simulink model "stewartpid_simulink"  (R2021b)
settings: Solver=FixedStepAuto  StartTime=0.0  StopTime=10.0  FixedStep=0.001  RelTol=1e-3
values from neighbouring files (symbols this model uses):
  contact = 0.05    [runthis.m]
  downMass = 0.1    [runthis.m]
  Kd = 0    [runthis.m]
  Ki = 0    [runthis.m]
  Kp = 0    [runthis.m]
  l1 = 0.35    [runthis.m]
  upMass = 0.1    [runthis.m]
undefined symbols (not defined in the file or in its folder): X, Y, Z
libraries: sm_lib x96, nesl_utility x30, slpidlib x1, sharedtransform x1
(part 1 of 3)
settings Model: Creator=Hitsz  LastModifiedBy=Hitsz

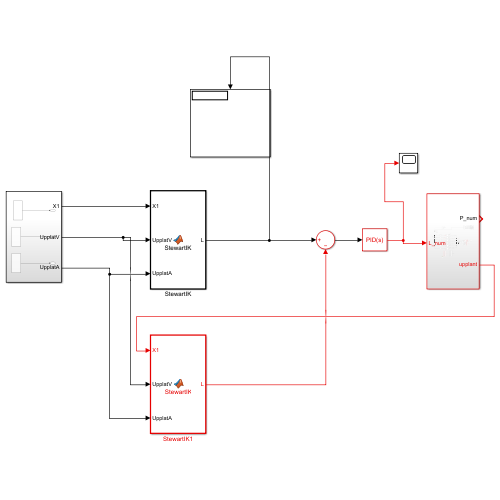
[thumbnail: Simulink's stored preview of the top-level diagram]
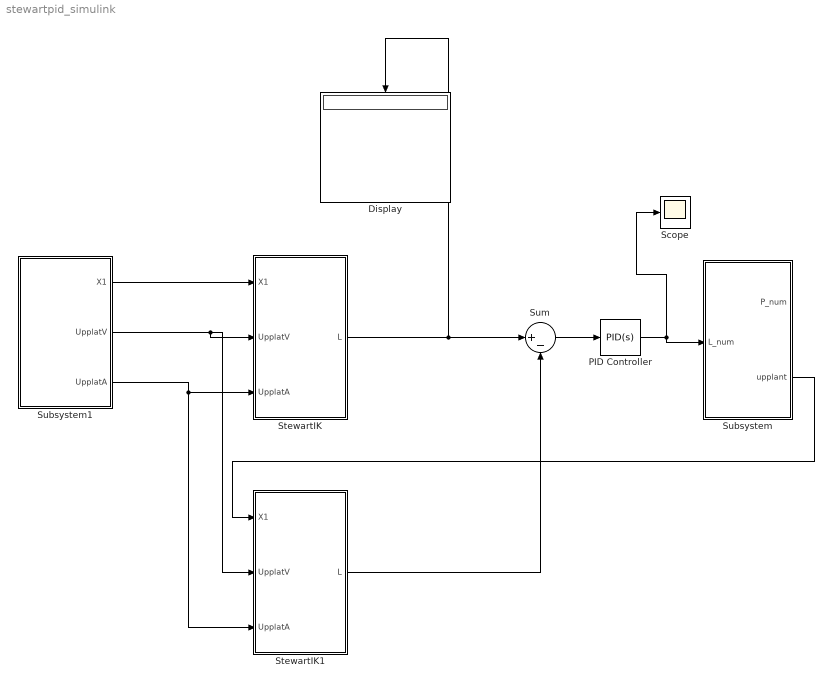
== system stewartpid_simulink ==
  Display : Display
  PID Controller : slpidlib/PID Controller  Controller=PID  Form=Parallel  TimeDomain=Continuous-time  UseExternalTs=off  SampleTime=-1  IntegratorMethod=Forward Euler  FilterMethod=Forward Euler  ControllerParametersSource=internal  P=Kp  I=Ki  D=Kd  UseFilter=on  N=100  TunerSelectOption=Transfer Function Based (PID Tuner App)  InitialConditionSource=internal  InitialConditionForIntegrator=0  InitialConditionForFilter=0  DifferentiatorICPrevScaledInput=0  ExternalReset=none  TrackingMode=off  Kt=1  LimitOutput=off  SatLimitsSource=internal  UpperSaturationLimit=inf  LowerSaturationLimit=-inf  LinearizeAsGain=on  AntiWindupMode=none  Kb=1  POutMin=[]  POutMax=[]  IOutMin=[]  IOutMax=[]  DOutMin=[]  DOutMax=[]  NOutMin=[]  NOutMax=[]  SumOutMin=[]  SumOutMax=[]  SaturationOutMin=[]  SaturationOutMax=[]  PParamMin=[]  PParamMax=[]  IParamMin=[]  IParamMax=[]  DParamMin=[]  DParamMax=[]  NParamMin=[]  NParamMax=[]  KbParamMin=[]  KbParamMax=[]  KtParamMin=[]  KtParamMax=[]  KbOutMin=[]  KbOutMax=[]  KtOutMin=[]  KtOutMax=[]  IntegratorOutMin=[]  IntegratorOutMax=[]  FilterOutMin=[]  FilterOutMax=[]  SumI1OutMin=[]  SumI1OutMax=[]  SumI2OutMin=[]  SumI2OutMax=[]  SumI3OutMin=[]  SumI3OutMax=[]  SumI4OutMin=[]  SumI4OutMax=[]  SumDOutMin=[]  SumDOutMax=[]  DifferentiatorOutMin=[]  DifferentiatorOutMax=[]  FilterDiffOutCoefMin=[]  FilterDiffOutCoefMax=[]  ReciprocalOutMin=[]  ReciprocalOutMax=[]  SumDenOutMin=[]  SumDenOutMax=[]  SumNumOutMin=[]  SumNumOutMax=[]  DivideOutMin=[]  DivideOutMax=[]  UdiffTsProdOutMin=[]  UdiffTsProdOutMax=[]  NTsProdOutMin=[]  NTsProdOutMax=[]  UintegralTsProdOutMin=[]  UintegralTsProdOutMax=[]  UngainTsProdOutMin=[]  UngainTsProdOutMax=[]  IntegratorContinuousStateAttributes=''  IntegratorStateMustResolveToSignalObject=off  IntegratorRTWStateStorageClass=Auto  FilterContinuousStateAttributes=''  FilterStateMustResolveToSignalObject=off  FilterRTWStateStorageClass=Auto  ParallelPVariant=InternalParameters  IdealPVariant=Disabled  IVariant=InternalParameters  DVariant=InternalParameters  IntegratorVariant=Continuous  SatVariant=Disabled  AWVariant=Passthrough  PCopyVariant=Disabled  TRVariant=Disabled  FdbkBlocksVariant=Forward  IdealPFdbkVariant=Disabled  SatFdbkVariant=Disabled  DerivativeFilterVariant=ContFilter  NVariant=InternalParameters  NCopyVariant=Disabled  FilterICVariant=InternalICsFilter  IntegratorICVariant=InternalICs  ExternalResetVariant=Disabled  TRSumVariant=Passthrough  SumFdbkVariant=Disabled  SumVariant=Sum_PID  TsampFilterVariant=InternalTs  TsampNgainVariant=Passthrough  TsampIntegralVariant=Passthrough  ExternalSaturationOutDataTypeStr=Inherit: Same as second input
  Scope : Scope
  StewartIK : MATLAB Function  TreatAsAtomicUnit=on
  StewartIK1 : MATLAB Function  TreatAsAtomicUnit=on
  Subsystem : Subsystem
  Subsystem1 : Subsystem
  Sum : Sum  Inputs=|+-
  wires:
  Subsystem1/1(X1) -> StewartIK/1(X1)
  Subsystem1/2(UpplatV) -> StewartIK1/2(UpplatV), StewartIK/2(UpplatV)
  Subsystem1/3(UpplatA) -> StewartIK1/3(UpplatA), StewartIK/3(UpplatA)
  StewartIK/1(L) -> Sum/1, Display/1
  Sum/1 -> PID Controller/1
  PID Controller/1 -> Scope/1, Subsystem/1(L_num)
  Subsystem/2(upplant) -> StewartIK1/1(X1)
  StewartIK1/1(L) -> Sum/2

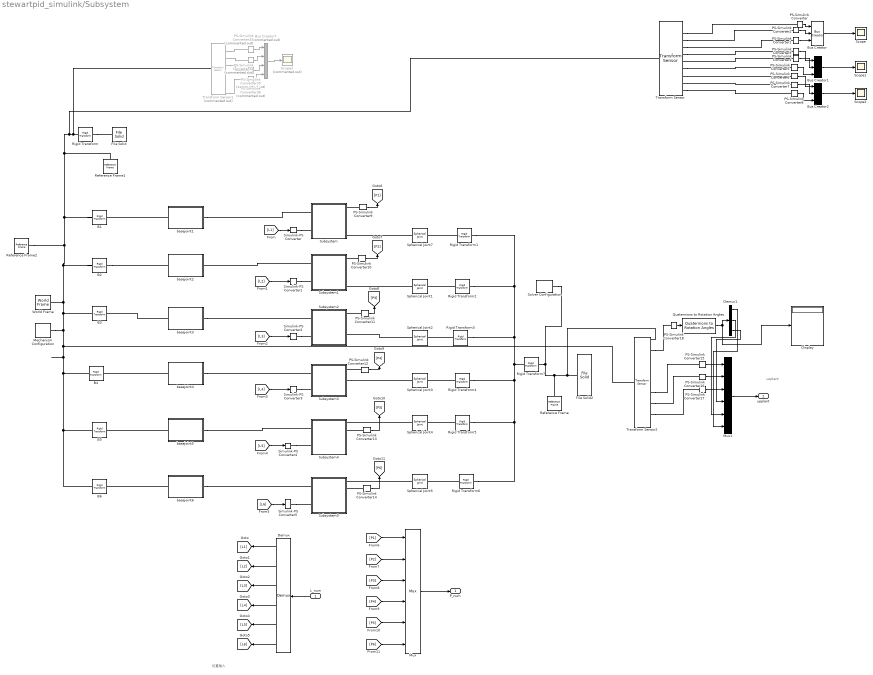
== system stewartpid_simulink/Subsystem ==
  note: uoplant
  note: 位置输入
  L_num : Inport
  "B1 " : sm_lib/Frames and Transforms/Rigid Transform  TranslationMethod=Cartesian  TranslationStandardOffset=0  TranslationLengthUnit=m  TranslationStandardAxis=+Z  TranslationCartesianOffset=B1  TranslationROffset=0  TranslationROffsetUnits=m  TranslationZOffset=0  TranslationZOffsetUnits=m  TranslationThetaOffset=0  TranslationThetaOffsetUnits=deg  RotationMethod=None  RotationAngleUnits=deg  RotationStandardAxis=+Z  RotationAngle=0.0  RotationArbitraryAxis=[0 0 1]  FollAlignAxisA=+X  BaseAlignAxisA=+Y  FollAlignAxisB=+Y  BaseAlignAxisB=+Z  RotationSequenceAxes=FollowerAxes  RotationSequence=XYX  RotationSequenceAngles=[0 0 0]  RotationSequenceAnglesUnits=deg  RotationMatrix=[1 0 0; 0 1 0; 0 0 1]
  "B2 " : sm_lib/Frames and Transforms/Rigid Transform  TranslationMethod=Cartesian  TranslationStandardOffset=0  TranslationLengthUnit=m  TranslationStandardAxis=+Z  TranslationCartesianOffset=B2  TranslationROffset=0  TranslationROffsetUnits=m  TranslationZOffset=0  TranslationZOffsetUnits=m  TranslationThetaOffset=0  TranslationThetaOffsetUnits=deg  RotationMethod=None  RotationAngleUnits=deg  RotationStandardAxis=+Z  RotationAngle=0.0  RotationArbitraryAxis=[0 0 1]  FollAlignAxisA=+X  BaseAlignAxisA=+Y  FollAlignAxisB=+Y  BaseAlignAxisB=+Z  RotationSequenceAxes=FollowerAxes  RotationSequence=XYX  RotationSequenceAngles=[0 0 0]  RotationSequenceAnglesUnits=deg  RotationMatrix=[1 0 0; 0 1 0; 0 0 1]
  "B3 " : sm_lib/Frames and Transforms/Rigid Transform  TranslationMethod=Cartesian  TranslationStandardOffset=0  TranslationLengthUnit=m  TranslationStandardAxis=+Z  TranslationCartesianOffset=B3  TranslationROffset=0  TranslationROffsetUnits=m  TranslationZOffset=0  TranslationZOffsetUnits=m  TranslationThetaOffset=0  TranslationThetaOffsetUnits=deg  RotationMethod=None  RotationAngleUnits=deg  RotationStandardAxis=+Z  RotationAngle=0.0  RotationArbitraryAxis=[0 0 1]  FollAlignAxisA=+X  BaseAlignAxisA=+Y  FollAlignAxisB=+Y  BaseAlignAxisB=+Z  RotationSequenceAxes=FollowerAxes  RotationSequence=XYX  RotationSequenceAngles=[0 0 0]  RotationSequenceAnglesUnits=deg  RotationMatrix=[1 0 0; 0 1 0; 0 0 1]
  "B4 " : sm_lib/Frames and Transforms/Rigid Transform  TranslationMethod=Cartesian  TranslationStandardOffset=0  TranslationLengthUnit=m  TranslationStandardAxis=+Z  TranslationCartesianOffset=B4  TranslationROffset=0  TranslationROffsetUnits=m  TranslationZOffset=0  TranslationZOffsetUnits=m  TranslationThetaOffset=0  TranslationThetaOffsetUnits=deg  RotationMethod=None  RotationAngleUnits=deg  RotationStandardAxis=+Z  RotationAngle=0.0  RotationArbitraryAxis=[0 0 1]  FollAlignAxisA=+X  BaseAlignAxisA=+Y  FollAlignAxisB=+Y  BaseAlignAxisB=+Z  RotationSequenceAxes=FollowerAxes  RotationSequence=XYX  RotationSequenceAngles=[0 0 0]  RotationSequenceAnglesUnits=deg  RotationMatrix=[1 0 0; 0 1 0; 0 0 1]
  "B5 " : sm_lib/Frames and Transforms/Rigid Transform  TranslationMethod=Cartesian  TranslationStandardOffset=0  TranslationLengthUnit=m  TranslationStandardAxis=+Z  TranslationCartesianOffset=B5  TranslationROffset=0  TranslationROffsetUnits=m  TranslationZOffset=0  TranslationZOffsetUnits=m  TranslationThetaOffset=0  TranslationThetaOffsetUnits=deg  RotationMethod=None  RotationAngleUnits=deg  RotationStandardAxis=+Z  RotationAngle=0.0  RotationArbitraryAxis=[0 0 1]  FollAlignAxisA=+X  BaseAlignAxisA=+Y  FollAlignAxisB=+Y  BaseAlignAxisB=+Z  RotationSequenceAxes=FollowerAxes  RotationSequence=XYX  RotationSequenceAngles=[0 0 0]  RotationSequenceAnglesUnits=deg  RotationMatrix=[1 0 0; 0 1 0; 0 0 1]
  "B6 " : sm_lib/Frames and Transforms/Rigid Transform  TranslationMethod=Cartesian  TranslationStandardOffset=0  TranslationLengthUnit=m  TranslationStandardAxis=+Z  TranslationCartesianOffset=B6  TranslationROffset=0  TranslationROffsetUnits=m  TranslationZOffset=0  TranslationZOffsetUnits=m  TranslationThetaOffset=0  TranslationThetaOffsetUnits=deg  RotationMethod=None  RotationAngleUnits=deg  RotationStandardAxis=+Z  RotationAngle=0.0  RotationArbitraryAxis=[0 0 1]  FollAlignAxisA=+X  BaseAlignAxisA=+Y  FollAlignAxisB=+Y  BaseAlignAxisB=+Z  RotationSequenceAxes=FollowerAxes  RotationSequence=XYX  RotationSequenceAngles=[0 0 0]  RotationSequenceAnglesUnits=deg  RotationMatrix=[1 0 0; 0 1 0; 0 0 1]
  Bus Creator : BusCreator  Inputs=3
  Bus Creator1 : BusCreator  Inputs=3
  Bus Creator2 : BusCreator  Inputs=3
  Bus Creator7 : BusCreator  Commented=on  Inputs=4
  Demux : Demux  Outputs=6
  Demux1 : Demux  Outputs=3
  Display : Display
  File Solid : sm_lib/Body Elements/File Solid  ExtGeomFileName=E:\onedrive\stewart_system\3_6_redundant\matlab_code\verification\verificationWithTraditionalControl\DOWN.STEP  UnitType=FromFile  ExtGeomFileUnits=m  StepReaderType=HEX  ExportConvexHullGeometry=off  InertiaType=Custom  Mass=1  MassUnits=kg  CenterOfMass=[0 0 0]  CenterOfMassUnits=m  MomentsOfInertia=[1 1 1]  MomentsOfInertiaUnits=kg*m^2  ProductsOfInertia=[0 0 0]  ProductsOfInertiaUnits=kg*m^2  BasedOnType=DensityFromFile  Density=1000  DensityUnits=kg/m^3  DoExposeReferenceFrame=off  SerializedFrames=<Frames><Frame><Id>Frame1</Id><Value><Name>F1</Name><Origin><Source>ReferenceFrame</Source><FeatureName></FeatureName></Origin><PrimaryAxis><DefinedDirection>+Z</DefinedDirection><Source>ReferenceFrame</Source><SourceDirection>+Z</SourceDirection><FeatureName></FeatureName></PrimaryAxis><SecondaryAxis><DefinedDirection>+X</DefinedDirection><Source>ReferenceFrame</Source><SourceDirection>+X</SourceDirection><FeatureName></FeatureName></SecondaryAxis></Value></Frame></Frames>  GraphicType=FromGeometry  MarkerShape=Sphere  MarkerSize=10  GraphicVisPropType=SimpleVisualProperties  GraphicDiffuseColor=[0.8 0.8 0.0]  GraphicSpecularColor=[0.5 0.5 0.5 1.0]  GraphicAmbientColor=[0.15 0.15 0.15 1.0]  GraphicEmissiveColor=[0.0 0.0 0.0 1.0]  GraphicShininess=75  GraphicOpacity=1.0
  File Solid2 : sm_lib/Body Elements/File Solid  ExtGeomFileName=E:\onedrive\stewart_system\3_6_redundant\matlab_code\verification\verificationWithTraditionalControl\UP.STEP  UnitType=FromFile  ExtGeomFileUnits=m  StepReaderType=HEX  ExportConvexHullGeometry=off  InertiaType=Custom  Mass=1.5  MassUnits=kg  CenterOfMass=[0 0 0]  CenterOfMassUnits=m  MomentsOfInertia=[0.08 0.08 .08]  MomentsOfInertiaUnits=kg*m^2  ProductsOfInertia=[0 0 0]  ProductsOfInertiaUnits=kg*m^2  BasedOnType=DensityFromFile  Density=1000  DensityUnits=kg/m^3  DoExposeReferenceFrame=off  SerializedFrames=<Frames><Frame><Id>Frame1</Id><Value><Name>M0</Name><Origin><Source>ReferenceFrame</Source><FeatureName></FeatureName></Origin><PrimaryAxis><DefinedDirection>+Z</DefinedDirection><Source>ReferenceFrame</Source><SourceDirection>+Z</SourceDirection><FeatureName></FeatureName></PrimaryAxis><SecondaryAxis><DefinedDirection>+X</DefinedDirection><Source>ReferenceFrame</Source><SourceDirection>+X</SourceDirection><FeatureName></FeatureName></SecondaryAxis></Value></Frame></Frames>  GraphicType=FromGeometry  MarkerShape=Sphere  MarkerSize=10  GraphicVisPropType=SimpleVisualProperties  GraphicDiffuseColor=[1.0 0.0 0.8]  GraphicSpecularColor=[0.5 0.5 0.5 1.0]  GraphicAmbientColor=[0.15 0.15 0.15 1.0]  GraphicEmissiveColor=[0.0 0.0 0.0 1.0]  GraphicShininess=75  GraphicOpacity=1.0
  Mechanism Configuration : sm_lib/Utilities/Mechanism Configuration  UniformGravity=Constant  GravityVector=[0 0 -9.807]  GravityUnits=m/s^2  LinearizationDelta=0.001  JointModeTransitionNonlinearIterations=2
  Mux : Mux  Inputs=6
  Mux1 : Mux  Inputs=6
  PS-Simulink Converter{,1..18} (19 alike) : nesl_utility/PS-Simulink Converter  PhysicalDomain=network_engine_domain  SubClassName=ps_output  LeftPortType=input  RightPortType=output  PseudoPeriodic=off  Frequencies=[]  Unit=inherit  AffineConversion=off
      settings: SourceProductBaseCode=PW,SS
  PS-Simulink Converter{33..36} (4 alike) : nesl_utility/PS-Simulink Converter  Commented=on  PhysicalDomain=network_engine_domain  SubClassName=ps_output  LeftPortType=input  RightPortType=output  PseudoPeriodic=off  Frequencies=[]  Unit=inherit  AffineConversion=off
      settings: SourceProductBaseCode=PW,SS
  Quaternions to Rotation Angles : sharedtransform/Quaternions to Rotation Angles  rotationOrder=ZYX  aMode=aMode
      settings: SourceProductBaseCode=AE,PW,DR,MT,UV,VE
  Reference Frame : sm_lib/Frames and Transforms/Reference Frame
  Reference Frame1 : sm_lib/Frames and Transforms/Reference Frame
  Reference Frame2 : sm_lib/Frames and Transforms/Reference Frame
  Rigid Transform : sm_lib/Frames and Transforms/Rigid Transform  TranslationMethod=None  TranslationStandardOffset=0  TranslationLengthUnit=m  TranslationStandardAxis=+Z  TranslationCartesianOffset=[0 0 0]  TranslationROffset=0  TranslationROffsetUnits=m  TranslationZOffset=0  TranslationZOffsetUnits=m  TranslationThetaOffset=0  TranslationThetaOffsetUnits=deg  RotationMethod=None  RotationAngleUnits=deg  RotationStandardAxis=+X  RotationAngle=90  RotationArbitraryAxis=[0 0 1]  FollAlignAxisA=+X  BaseAlignAxisA=+Y  FollAlignAxisB=+Y  BaseAlignAxisB=+Z  RotationSequenceAxes=FollowerAxes  RotationSequence=XYX  RotationSequenceAngles=[0 0 0]  RotationSequenceAnglesUnits=deg  RotationMatrix=[1 0 0; 0 1 0; 0 0 1]
  Rigid Transform1 : sm_lib/Frames and Transforms/Rigid Transform  TranslationMethod=Cartesian  TranslationStandardOffset=0  TranslationLengthUnit=m  TranslationStandardAxis=+Z  TranslationCartesianOffset=T1_Ti  TranslationROffset=0  TranslationROffsetUnits=m  TranslationZOffset=0  TranslationZOffsetUnits=m  TranslationThetaOffset=0  TranslationThetaOffsetUnits=deg  RotationMethod=None  RotationAngleUnits=deg  RotationStandardAxis=+Z  RotationAngle=0.0  RotationArbitraryAxis=[0 0 1]  FollAlignAxisA=+X  BaseAlignAxisA=+Y  FollAlignAxisB=+Y  BaseAlignAxisB=+Z  RotationSequenceAxes=FollowerAxes  RotationSequence=XYX  RotationSequenceAngles=[0 0 0]  RotationSequenceAnglesUnits=deg  RotationMatrix=[1 0 0; 0 1 0; 0 0 1]
  Rigid Transform2 : sm_lib/Frames and Transforms/Rigid Transform  TranslationMethod=Cartesian  TranslationStandardOffset=0  TranslationLengthUnit=m  TranslationStandardAxis=+Z  TranslationCartesianOffset=T2_Ti  TranslationROffset=0  TranslationROffsetUnits=m  TranslationZOffset=0  TranslationZOffsetUnits=m  TranslationThetaOffset=0  TranslationThetaOffsetUnits=deg  RotationMethod=None  RotationAngleUnits=deg  RotationStandardAxis=+Z  RotationAngle=0.0  RotationArbitraryAxis=[0 0 1]  FollAlignAxisA=+X  BaseAlignAxisA=+Y  FollAlignAxisB=+Y  BaseAlignAxisB=+Z  RotationSequenceAxes=FollowerAxes  RotationSequence=XYX  RotationSequenceAngles=[0 0 0]  RotationSequenceAnglesUnits=deg  RotationMatrix=[1 0 0; 0 1 0; 0 0 1]
  Rigid Transform3 : sm_lib/Frames and Transforms/Rigid Transform  TranslationMethod=Cartesian  TranslationStandardOffset=0  TranslationLengthUnit=m  TranslationStandardAxis=+Z  TranslationCartesianOffset=T3_Ti  TranslationROffset=0  TranslationROffsetUnits=m  TranslationZOffset=0  TranslationZOffsetUnits=m  TranslationThetaOffset=0  TranslationThetaOffsetUnits=deg  RotationMethod=None  RotationAngleUnits=deg  RotationStandardAxis=+Z  RotationAngle=0.0  RotationArbitraryAxis=[0 0 1]  FollAlignAxisA=+X  BaseAlignAxisA=+Y  FollAlignAxisB=+Y  BaseAlignAxisB=+Z  RotationSequenceAxes=FollowerAxes  RotationSequence=XYX  RotationSequenceAngles=[0 0 0]  RotationSequenceAnglesUnits=deg  RotationMatrix=[1 0 0; 0 1 0; 0 0 1]
  Rigid Transform4 : sm_lib/Frames and Transforms/Rigid Transform  TranslationMethod=Cartesian  TranslationStandardOffset=0  TranslationLengthUnit=m  TranslationStandardAxis=+Z  TranslationCartesianOffset=T4_Ti  TranslationROffset=0  TranslationROffsetUnits=m  TranslationZOffset=0  TranslationZOffsetUnits=m  TranslationThetaOffset=0  TranslationThetaOffsetUnits=deg  RotationMethod=None  RotationAngleUnits=deg  RotationStandardAxis=+Z  RotationAngle=0.0  RotationArbitraryAxis=[0 0 1]  FollAlignAxisA=+X  BaseAlignAxisA=+Y  FollAlignAxisB=+Y  BaseAlignAxisB=+Z  RotationSequenceAxes=FollowerAxes  RotationSequence=XYX  RotationSequenceAngles=[0 0 0]  RotationSequenceAnglesUnits=deg  RotationMatrix=[1 0 0; 0 1 0; 0 0 1]
  Rigid Transform5 : sm_lib/Frames and Transforms/Rigid Transform  TranslationMethod=Cartesian  TranslationStandardOffset=0  TranslationLengthUnit=m  TranslationStandardAxis=+Z  TranslationCartesianOffset=T5_Ti  TranslationROffset=0  TranslationROffsetUnits=m  TranslationZOffset=0  TranslationZOffsetUnits=m  TranslationThetaOffset=0  TranslationThetaOffsetUnits=deg  RotationMethod=None  RotationAngleUnits=deg  RotationStandardAxis=+Z  RotationAngle=0.0  RotationArbitraryAxis=[0 0 1]  FollAlignAxisA=+X  BaseAlignAxisA=+Y  FollAlignAxisB=+Y  BaseAlignAxisB=+Z  RotationSequenceAxes=FollowerAxes  RotationSequence=XYX  RotationSequenceAngles=[0 0 0]  RotationSequenceAnglesUnits=deg  RotationMatrix=[1 0 0; 0 1 0; 0 0 1]
  Rigid Transform6 : sm_lib/Frames and Transforms/Rigid Transform  TranslationMethod=Cartesian  TranslationStandardOffset=0  TranslationLengthUnit=m  TranslationStandardAxis=+Z  TranslationCartesianOffset=T6_Ti  TranslationROffset=0  TranslationROffsetUnits=m  TranslationZOffset=0  TranslationZOffsetUnits=m  TranslationThetaOffset=0  TranslationThetaOffsetUnits=deg  RotationMethod=None  RotationAngleUnits=deg  RotationStandardAxis=+Z  RotationAngle=0.0  RotationArbitraryAxis=[0 0 1]  FollAlignAxisA=+X  BaseAlignAxisA=+Y  FollAlignAxisB=+Y  BaseAlignAxisB=+Z  RotationSequenceAxes=FollowerAxes  RotationSequence=XYX  RotationSequenceAngles=[0 0 0]  RotationSequenceAnglesUnits=deg  RotationMatrix=[1 0 0; 0 1 0; 0 0 1]
  Rigid Transform7 : sm_lib/Frames and Transforms/Rigid Transform  TranslationMethod=None  TranslationStandardOffset=0  TranslationLengthUnit=m  TranslationStandardAxis=+Z  TranslationCartesianOffset=[0 0 0]  TranslationROffset=0  TranslationROffsetUnits=m  TranslationZOffset=0  TranslationZOffsetUnits=m  TranslationThetaOffset=0  TranslationThetaOffsetUnits=deg  RotationMethod=StandardAxis  RotationAngleUnits=deg  RotationStandardAxis=+Z  RotationAngle=180  RotationArbitraryAxis=[0 0 1]  FollAlignAxisA=+X  BaseAlignAxisA=+Y  FollAlignAxisB=+Y  BaseAlignAxisB=+Z  RotationSequenceAxes=FollowerAxes  RotationSequence=XYX  RotationSequenceAngles=[0 0 0]  RotationSequenceAnglesUnits=deg  RotationMatrix=[1 0 0; 0 1 0; 0 0 1]
  Scope : Scope
  Scope1 : Scope
  Scope2 : Scope
  Scope3 : Scope  Commented=on
  Simulink-PS Converter{,1..5} (6 alike) : nesl_utility/Simulink-PS Converter  PhysicalDomain=network_engine_domain  SubClassName=ps_input  LeftPortType=input  RightPortType=output  PseudoPeriodic=off  Frequencies=[]  NoiseDistribution=none  NoiseParameters=[]  Unit=1  AffineConversion=off  FilteringAndDerivatives=filter  SimscapeFilterOrder=2  InputFilterTimeConstant=0.001  UdotUserProvided=0
      settings: SourceProductBaseCode=PW,SS
  Solver Configuration : nesl_utility/Solver Configuration  PhysicalDomain=network_engine_domain  SubClassName=solver  LeftPortType=input  RightPortType=generic  Tones=[]  Harmonics=[]  SimulateNoise=off  Profile=off  UseLocalSampling=off  EnableSwitchedLinearOptims=on  FrequencyDomain=off  UseCCode=off  RelTol=0.001  AbsTol=1e-06  MinStep=1e-09  ToWorkspace=off  RevertToSquareIcSolve=off  NumHomotopyIterations=100  PhasorMode=off  PhasorModeNumHarmonics=1  DoDC=off  ResidualTolerance=1e-09  UseLocalSolver=off  LocalSolverChoice=NE_TRAPEZOIDAL_ADVANCER  LocalSolverSampleTime=0.001  DoFixedCost=off  MaxNonlinIter=3  MaxModeIter=2  ComputeImpulses=off  ImpulseIterations=2  LinearAlgebra=Sparse  EquationFormulation=NE_FREQUENCY_TIME_EF  DelaysMemoryBudget=1024  AutomaticFiltering=off  FilteringTimeConstant=0.001  PartitionStorageMethod=AS_NEEDED  PartitionMemoryBudget=1024  PartitionMethod=ROBUST
      settings: SourceProductBaseCode=PW,SS
  Spherical Joint{1..4,7} (5 alike) : sm_lib/Joints/Spherical Joint  JointMode=Normal  SenseConstraintForce=off  SenseConstraintForceX=off  SenseConstraintForceY=off  SenseConstraintForceZ=off  SenseConstraintTorque=off  SenseConstraintTorqueX=off  SenseConstraintTorqueY=off  SenseConstraintTorqueZ=off  SenseTotalForce=off  SenseTotalForceX=off  SenseTotalForceY=off  SenseTotalForceZ=off  SenseTotalTorque=off  SenseTotalTorqueX=off  SenseTotalTorqueY=off  SenseTotalTorqueZ=off  CompositeWrenchDir=FollowerOnBase  CompositeWrenchFrame=BaseFrame  DefPosRotationMethod=None  DefPosRotationAngleUnits=deg  DefPosRotationStandardAxis=+Z  DefPosRotationAngle=0.0  DefPosRotationArbitraryAxis=[0 0 1]  DefPosFollAlignAxisA=+X  DefPosBaseAlignAxisA=+Y  DefPosFollAlignAxisB=+Y  DefPosBaseAlignAxisB=+Z  DefPosRotationSequenceAxes=FollowerAxes  DefPosRotationSequence=XYX  DefPosRotationSequenceAngles=[0 0 0]  DefPosRotationSequenceAnglesUnits=deg  DefPosRotationMatrix=[1 0 0; 0 1 0; 0 0 1]  EqPosRotationMethod=None  EqPosRotationAngleUnits=deg  EqPosRotationStandardAxis=+Z  EqPosRotationAngle=0.0  EqPosRotationArbitraryAxis=[0 0 1]  EqPosFollAlignAxisA=+X  EqPosBaseAlignAxisA=+Y  EqPosFollAlignAxisB=+Y  EqPosBaseAlignAxisB=+Z  EqPosRotationSequenceAxes=FollowerAxes  EqPosRotationSequence=XYX  EqPosRotationSequenceAngles=[0 0 0]  EqPosRotationSequenceAnglesUnits=deg  EqPosRotationMatrix=[1 0 0; 0 1 0; 0 0 1]  SpringStiffness=0  SpringStiffnessUnits=N*m/deg  DampingCoefficient=0  DampingCoefficientUnits=N*m/(deg/s)  ActuateTorqueX=off  ActuateTorqueY=off  ActuateTorqueZ=off  ActuateTorque=off  TorqueActuationMode=NoTorque  MotionActuationMode=ComputedMotion  ActuationFrame=BaseFrame  SensePosition=off  SenseVelocityX=off  SenseVelocityY=off  SenseVelocityZ=off  SenseVelocity=off  SenseAccelerationX=off  SenseAccelerationY=off  SenseAccelerationZ=off  SenseAcceleration=off  SenseTorqueX=off  SenseTorqueY=off  SenseTorqueZ=off  SenseTorqueForce=off  SenseLowerLimitTorqueMag=off  SenseUpperLimitTorqueMag=off  SensingFrame=BaseFrame  LowerLimitSpecify=on  LowerLimitBound=spheredown  LowerLimitBoundUnits=deg  LowerLimitStiffness=sprsti  LowerLimitStiffnessUnits=N*m/deg  LowerLimitDamping=damcoe  LowerLimitDampingUnits=N*m/(deg/s)  LowerLimitTransitionRegionWidth=trare  LowerLimitTransitionRegionWidthUnits=deg  UpperLimitSpecify=on  UpperLimitBound=sphereup  UpperLimitBoundUnits=deg  UpperLimitStiffness=sprsti  UpperLimitStiffnessUnits=N*m/deg  UpperLimitDamping=damcoe  UpperLimitDampingUnits=N*m/(deg/s)  UpperLimitTransitionRegionWidth=trare  UpperLimitTransitionRegionWidthUnits=deg  PositionTargetRotationMethod=None  PositionTargetRotationAngleUnits=deg  PositionTargetRotationStandardAxis=+Z  PositionTargetRotationAngle=0.0  PositionTargetRotationArbitraryAxis=[0 0 1]  PositionTargetFollAlignAxisA=+X  PositionTargetBaseAlignAxisA=+Y  PositionTargetFollAlignAxisB=+Y  PositionTargetBaseAlignAxisB=+Z  PositionTargetRotationSequenceAxes=FollowerAxes  PositionTargetRotationSequence=XYX  PositionTargetRotationSequenceAngles=[0 0 0]  PositionTargetRotationSequenceAnglesUnits=deg  PositionTargetRotationMatrix=[1 0 0; 0 1 0; 0 0 1]  PositionTargetSpecify=off  PositionTargetPriority=High  VelocityTargetValue=[0 0 0]  VelocityTargetValueUnits=deg/s  VelocityTargetSpecify=off  VelocityTargetPriority=High  VelocityTargetInFollowerFrame=on
  Spherical Joint5 : sm_lib/Joints/Spherical Joint  JointMode=Normal  SenseConstraintForce=off  SenseConstraintForceX=off  SenseConstraintForceY=off  SenseConstraintForceZ=off  SenseConstraintTorque=off  SenseConstraintTorqueX=off  SenseConstraintTorqueY=off  SenseConstraintTorqueZ=off  SenseTotalForce=off  SenseTotalForceX=off  SenseTotalForceY=off  SenseTotalForceZ=off  SenseTotalTorque=off  SenseTotalTorqueX=off  SenseTotalTorqueY=off  SenseTotalTorqueZ=off  CompositeWrenchDir=FollowerOnBase  CompositeWrenchFrame=BaseFrame  DefPosRotationMethod=None  DefPosRotationAngleUnits=deg  DefPosRotationStandardAxis=+Z  DefPosRotationAngle=0.0  DefPosRotationArbitraryAxis=[0 0 1]  DefPosFollAlignAxisA=+X  DefPosBaseAlignAxisA=+Y  DefPosFollAlignAxisB=+Y  DefPosBaseAlignAxisB=+Z  DefPosRotationSequenceAxes=FollowerAxes  DefPosRotationSequence=XYX  DefPosRotationSequenceAngles=[0 0 0]  DefPosRotationSequenceAnglesUnits=deg  DefPosRotationMatrix=[1 0 0; 0 1 0; 0 0 1]  EqPosRotationMethod=None  EqPosRotationAngleUnits=deg  EqPosRotationStandardAxis=+Z  EqPosRotationAngle=0.0  EqPosRotationArbitraryAxis=[0 0 1]  EqPosFollAlignAxisA=+X  EqPosBaseAlignAxisA=+Y  EqPosFollAlignAxisB=+Y  EqPosBaseAlignAxisB=+Z  EqPosRotationSequenceAxes=FollowerAxes  EqPosRotationSequence=XYX  EqPosRotationSequenceAngles=[0 0 0]  EqPosRotationSequenceAnglesUnits=deg  EqPosRotationMatrix=[1 0 0; 0 1 0; 0 0 1]  SpringStiffness=0  SpringStiffnessUnits=N*m/deg  DampingCoefficient=0  DampingCoefficientUnits=N*m/(deg/s)  ActuateTorqueX=off  ActuateTorqueY=off  ActuateTorqueZ=off  ActuateTorque=off  TorqueActuationMode=NoTorque  MotionActuationMode=ComputedMotion  ActuationFrame=BaseFrame  SensePosition=off  SenseVelocityX=off  SenseVelocityY=off  SenseVelocityZ=off  SenseVelocity=off  SenseAccelerationX=off  SenseAccelerationY=off  SenseAccelerationZ=off  SenseAcceleration=off  SenseTorqueX=off  SenseTorqueY=off  SenseTorqueZ=off  SenseTorqueForce=off  SenseLowerLimitTorqueMag=off  SenseUpperLimitTorqueMag=off  SensingFrame=BaseFrame  LowerLimitSpecify=off  LowerLimitBound=spheredown  LowerLimitBoundUnits=deg  LowerLimitStiffness=sprsti  LowerLimitStiffnessUnits=N*m/deg  LowerLimitDamping=damcoe  LowerLimitDampingUnits=N*m/(deg/s)  LowerLimitTransitionRegionWidth=trare  LowerLimitTransitionRegionWidthUnits=deg  UpperLimitSpecify=off  UpperLimitBound=sphereup  UpperLimitBoundUnits=deg  UpperLimitStiffness=sprsti  UpperLimitStiffnessUnits=N*m/deg  UpperLimitDamping=damcoe  UpperLimitDampingUnits=N*m/(deg/s)  UpperLimitTransitionRegionWidth=trare  UpperLimitTransitionRegionWidthUnits=deg  PositionTargetRotationMethod=None  PositionTargetRotationAngleUnits=deg  PositionTargetRotationStandardAxis=+Z  PositionTargetRotationAngle=0.0  PositionTargetRotationArbitraryAxis=[0 0 1]  PositionTargetFollAlignAxisA=+X  PositionTargetBaseAlignAxisA=+Y  PositionTargetFollAlignAxisB=+Y  PositionTargetBaseAlignAxisB=+Z  PositionTargetRotationSequenceAxes=FollowerAxes  PositionTargetRotationSequence=XYX  PositionTargetRotationSequenceAngles=[0 0 0]  PositionTargetRotationSequenceAnglesUnits=deg  PositionTargetRotationMatrix=[1 0 0; 0 1 0; 0 0 1]  PositionTargetSpecify=off  PositionTargetPriority=High  VelocityTargetValue=[0 0 0]  VelocityTargetValueUnits=deg/s  VelocityTargetSpecify=off  VelocityTargetPriority=High  VelocityTargetInFollowerFrame=on
  Subsystem : Subsystem
  Subsystem1 : Subsystem
  Subsystem2 : Subsystem
  Subsystem3 : Subsystem
  Subsystem4 : Subsystem
  Subsystem5 : Subsystem
  Transform Sensor : sm_lib/Frames and Transforms/Transform Sensor  MeasurementFrame=World  SenseAngle=off  SenseAxis=off  SenseAngle1=off  SenseAngle2=off  SenseAngle3=off  SenseQ=off  SenseR=off  SenseOmegaX=off  SenseOmegaY=off  SenseOmegaZ=off  SenseOmega1=off  SenseOmega2=off  SenseOmega3=off  SenseQDot=off  SenseRDot=off  SenseAlphaX=off  SenseAlphaY=off  SenseAlphaZ=off  SenseAlpha1=off  SenseAlpha2=off  SenseAlpha3=off  SenseQDDot=off  SenseRDDot=off  SenseX=on  SenseY=on  SenseZ=on  SenseRad=off  SenseAzim=off  SenseDist=off  SenseInc=off  SenseXDot=on  SenseYDot=on  SenseZDot=on  SenseRadDot=off  SenseAzimDot=off  SenseDistDot=off  SenseIncDot=off  SenseXDDot=on  SenseYDDot=on  SenseZDDot=on  SenseRadDDot=off  SenseAzimDDot=off  SenseDistDDot=off  SenseIncDDot=off
  Transform Sensor1 : sm_lib/Frames and Transforms/Transform Sensor  Commented=on  MeasurementFrame=Base  SenseAngle=off  SenseAxis=off  SenseAngle1=off  SenseAngle2=off  SenseAngle3=off  SenseQ=off  SenseR=off  SenseOmegaX=on  SenseOmegaY=on  SenseOmegaZ=on  SenseOmega1=off  SenseOmega2=off  SenseOmega3=off  SenseQDot=off  SenseRDot=off  SenseAlphaX=off  SenseAlphaY=off  SenseAlphaZ=off  SenseAlpha1=off  SenseAlpha2=off  SenseAlpha3=off  SenseQDDot=off  SenseRDDot=off  SenseX=off  SenseY=off  SenseZ=off  SenseRad=off  SenseAzim=off  SenseDist=off  SenseInc=off  SenseXDot=on  SenseYDot=on  SenseZDot=on  SenseRadDot=on  SenseAzimDot=off  SenseDistDot=off  SenseIncDot=off  SenseXDDot=off  SenseYDDot=off  SenseZDDot=off  SenseRadDDot=off  SenseAzimDDot=off  SenseDistDDot=off  SenseIncDDot=off
  Transform Sensor2 : sm_lib/Frames and Transforms/Transform Sensor  MeasurementFrame=Base  SenseAngle=off  SenseAxis=off  SenseAngle1=off  SenseAngle2=off  SenseAngle3=off  SenseQ=on  SenseR=off  SenseOmegaX=on  SenseOmegaY=on  SenseOmegaZ=on  SenseOmega1=off  SenseOmega2=off  SenseOmega3=off  SenseQDot=off  SenseRDot=off  SenseAlphaX=off  SenseAlphaY=off  SenseAlphaZ=off  SenseAlpha1=off  SenseAlpha2=off  SenseAlpha3=off  SenseQDDot=off  SenseRDDot=off  SenseX=on  SenseY=on  SenseZ=on  SenseRad=off  SenseAzim=off  SenseDist=off  SenseInc=off  SenseXDot=off  SenseYDot=off  SenseZDot=off  SenseRadDot=on  SenseAzimDot=off  SenseDistDot=off  SenseIncDot=off  SenseXDDot=off  SenseYDDot=off  SenseZDDot=off  SenseRadDDot=off  SenseAzimDDot=off  SenseDistDDot=off  SenseIncDDot=off
  World Frame : sm_lib/Frames and Transforms/World Frame
  basejoint1 : Subsystem
  basejoint2 : Subsystem
  basejoint3 : Subsystem
  basejoint4 : Subsystem
  basejoint5 : Subsystem
  basejoint6 : Subsystem
  P_num : Outport
  upplant : Outport  Port=2
  wires:
  PS-Simulink Converter1/1 -> Bus Creator/3
  PS-Simulink Converter2/1 -> Bus Creator/2
  PS-Simulink Converter/1 -> Bus Creator/1
  Bus Creator/1 -> Scope/1
  PS-Simulink Converter3/1 -> Bus Creator1/1
  PS-Simulink Converter4/1 -> Bus Creator1/2
  PS-Simulink Converter5/1 -> Bus Creator1/3
  PS-Simulink Converter6/1 -> Bus Creator2/1
  PS-Simulink Converter7/1 -> Bus Creator2/2
  PS-Simulink Converter8/1 -> Bus Creator2/3
  Bus Creator1/1 -> Scope1/1
  Bus Creator2/1 -> Scope2/1
  PS-Simulink Converter33/1 -> Bus Creator7/1
  PS-Simulink Converter34/1 -> Bus Creator7/2
  PS-Simulink Converter35/1 -> Bus Creator7/3
  Bus Creator7/1 -> Scope3/1
  PS-Simulink Converter36/1 -> Bus Creator7/4
  Demux/1 -> [L1]
  [L1] -> Simulink-PS Converter/1
  [L2] -> Simulink-PS Converter1/1
  [L3] -> Simulink-PS Converter2/1
  [L4] -> Simulink-PS Converter3/1
  [L5] -> Simulink-PS Converter4/1
  [L6] -> Simulink-PS Converter5/1
  Demux/2 -> [L2]
  Demux/3 -> [L3]
  Demux/4 -> [L4]
  Demux/5 -> [L5]
  Demux/6 -> [L6]
  L_num/1 -> Demux/1
  PS-Simulink Converter9/1 -> [P1]
  PS-Simulink Converter10/1 -> [P2]
  PS-Simulink Converter11/1 -> [P3]
  PS-Simulink Converter12/1 -> [P4]
  PS-Simulink Converter13/1 -> [P5]
  PS-Simulink Converter14/1 -> [P6]
  [P1] -> Mux/1
  [P2] -> Mux/2
  [P3] -> Mux/3
  [P4] -> Mux/4
  [P5] -> Mux/5
  [P6] -> Mux/6
  Mux/1 -> P_num/1
  PS-Simulink Converter15/1 -> Mux1/1
  PS-Simulink Converter16/1 -> Mux1/2
  PS-Simulink Converter17/1 -> Mux1/3
  PS-Simulink Converter18/1 -> Quaternions to Rotation Angles/1
  Demux1/3 -> Mux1/4
  Demux1/2 -> Mux1/5
  Demux1/1 -> Mux1/6
  Quaternions to Rotation Angles/1 -> Display/1, Demux1/1
  Mux1/1 -> upplant/1
  connections:
  Transform Sensor/RConn4 -- PS-Simulink Converter1/LConn1
  Mechanism Configuration/RConn1 -- Transform Sensor2/LConn1 -- "B6 "/LConn1 -- "B5 "/LConn1 -- "B4 "/LConn1 -- "B3 "/LConn1 -- Reference Frame1/RConn1 -- Transform Sensor1/LConn1 -- Rigid Transform/LConn1 -- Transform Sensor/LConn1 -- "B1 "/LConn1 -- Reference Frame2/RConn1 -- "B2 "/LConn1 -- World Frame/RConn1
  Rigid Transform/RConn1 -- File Solid/LConn1
  Transform Sensor/RConn3 -- PS-Simulink Converter2/LConn1
  Transform Sensor/RConn2 -- PS-Simulink Converter/LConn1
  Transform Sensor/RConn5 -- PS-Simulink Converter3/LConn1
  PS-Simulink Converter4/LConn1 -- Transform Sensor/RConn6
  Transform Sensor/RConn7 -- PS-Simulink Converter5/LConn1
  PS-Simulink Converter6/LConn1 -- Transform Sensor/RConn8
  PS-Simulink Converter7/LConn1 -- Transform Sensor/RConn9
  Transform Sensor/RConn10 -- PS-Simulink Converter8/LConn1
  Transform Sensor1/RConn2 -- PS-Simulink Converter33/LConn1
  Transform Sensor1/RConn3 -- PS-Simulink Converter34/LConn1
  Transform Sensor1/RConn4 -- PS-Simulink Converter35/LConn1
  Transform Sensor1/RConn8 -- PS-Simulink Converter36/LConn1
  Spherical Joint7/LConn1 -- Subsystem/RConn5
  Simulink-PS Converter/RConn1 -- Subsystem/LConn2
  PS-Simulink Converter9/LConn1 -- Subsystem/RConn1
  Spherical Joint1/LConn1 -- Subsystem1/RConn5
  Simulink-PS Converter1/RConn1 -- Subsystem1/LConn2
  PS-Simulink Converter10/LConn1 -- Subsystem1/RConn1
  Spherical Joint2/LConn1 -- Subsystem2/RConn4
  Simulink-PS Converter2/RConn1 -- Subsystem2/LConn2
  PS-Simulink Converter11/LConn1 -- Subsystem2/RConn1
  Spherical Joint3/LConn1 -- Subsystem3/RConn3
  Simulink-PS Converter3/RConn1 -- Subsystem3/LConn2
  PS-Simulink Converter12/LConn1 -- Subsystem3/RConn1
  Spherical Joint4/LConn1 -- Subsystem4/RConn1
  Simulink-PS Converter4/RConn1 -- Subsystem4/LConn2
  PS-Simulink Converter13/LConn1 -- Subsystem4/RConn2
  Spherical Joint5/LConn1 -- Subsystem5/RConn1
  Simulink-PS Converter5/RConn1 -- Subsystem5/LConn2
  PS-Simulink Converter14/LConn1 -- Subsystem5/RConn2
  Subsystem1/LConn1 -- basejoint2/RConn1
  basejoint3/RConn1 -- Subsystem2/LConn1
  basejoint1/RConn1 -- Subsystem/LConn1
  basejoint1/LConn1 -- "B1 "/RConn1
  "B2 "/RConn1 -- basejoint2/LConn1
  basejoint3/LConn1 -- "B3 "/RConn1
  basejoint4/LConn1 -- "B4 "/RConn1
  basejoint4/RConn1 -- Subsystem3/LConn1
  basejoint5/RConn1 -- Subsystem4/LConn1
  basejoint5/LConn1 -- "B5 "/RConn1
  basejoint6/LConn1 -- "B6 "/RConn1
  basejoint6/RConn1 -- Subsystem5/LConn1
  Rigid Transform1/LConn1 -- Spherical Joint7/RConn1
  Rigid Transform2/LConn1 -- Spherical Joint1/RConn1
  Rigid Transform3/LConn1 -- Spherical Joint2/RConn1
  Rigid Transform5/LConn1 -- Spherical Joint4/RConn1
  Rigid Transform4/LConn1 -- Spherical Joint3/RConn1
  Rigid Transform6/LConn1 -- Spherical Joint5/RConn1
  Rigid Transform7/RConn1 -- Solver Configuration/RConn1 -- Reference Frame/RConn1 -- Transform Sensor2/RConn1 -- File Solid2/LConn1
  Transform Sensor2/RConn6 -- PS-Simulink Converter15/LConn1
  Transform Sensor2/RConn7 -- PS-Simulink Converter16/LConn1
  Transform Sensor2/RConn8 -- PS-Simulink Converter17/LConn1
  Transform Sensor2/RConn2 -- PS-Simulink Converter18/LConn1
  Rigid Transform1/RConn1 -- Rigid Transform3/RConn1 -- Rigid Transform6/RConn1 -- Rigid Transform5/RConn1 -- Rigid Transform4/RConn1 -- Rigid Transform7/LConn1 -- Rigid Transform2/RConn1

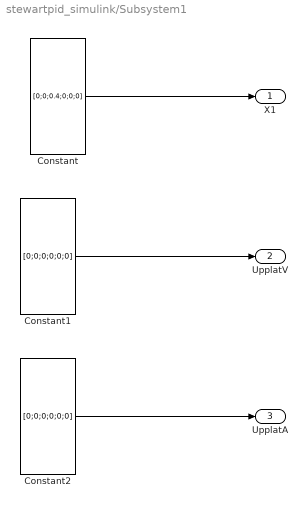
== system stewartpid_simulink/Subsystem1 ==
  Constant : Constant  Value=[0;0;0.4;0;0;0]  VectorParams1D=off
  Constant1 : Constant  Value=[0;0;0;0;0;0]  VectorParams1D=off
  Constant2 : Constant  Value=[0;0;0;0;0;0]  VectorParams1D=off
  X1 : Outport
  UpplatV : Outport  Port=2
  UpplatA : Outport  Port=3
  wires:
  Constant1/1 -> UpplatV/1
  Constant/1 -> X1/1
  Constant2/1 -> UpplatA/1

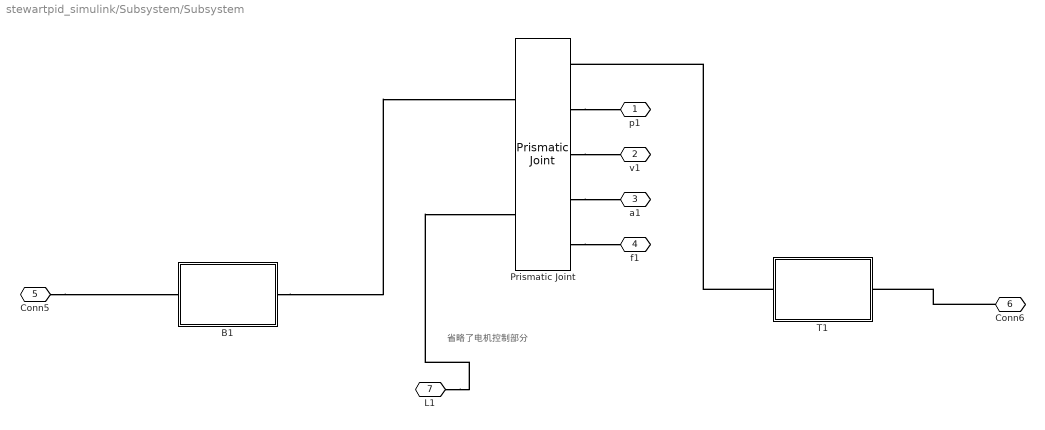
== system stewartpid_simulink/Subsystem/Subsystem ==
  note: 省略了电机控制部分
  "\tT1" : Subsystem
  B1 : Subsystem
  Prismatic Joint : sm_lib/Joints/Prismatic Joint  JointMode=Normal  SenseConstraintForce=off  SenseConstraintForceX=off  SenseConstraintForceY=off  SenseConstraintForceZ=off  SenseConstraintTorque=off  SenseConstraintTorqueX=off  SenseConstraintTorqueY=off  SenseConstraintTorqueZ=off  SenseTotalForce=off  SenseTotalForceX=off  SenseTotalForceY=off  SenseTotalForceZ=off  SenseTotalTorque=off  SenseTotalTorqueX=off  SenseTotalTorqueY=off  SenseTotalTorqueZ=off  CompositeWrenchDir=FollowerOnBase  CompositeWrenchFrame=BaseFrame  EquilibriumPosition=0  EquilibriumPositionUnits=m  SpringStiffness=0  SpringStiffnessUnits=N/m  DampingCoefficient=0  DampingCoefficientUnits=N/(m/s)  TorqueActuationMode=ComputedTorque  MotionActuationMode=InputMotion  SensePosition=on  SenseVelocity=on  SenseAcceleration=on  SenseTorqueForce=on  SenseLowerLimitTorqueForce=off  SenseUpperLimitTorqueForce=off  LowerLimitSpecify=on  LowerLimitBound=pingyilow  LowerLimitBoundUnits=m  LowerLimitStiffness=sprsti  LowerLimitStiffnessUnits=N/m  LowerLimitDamping=damcoe  LowerLimitDampingUnits=N/(m/s)  LowerLimitTransitionRegionWidth=trare  LowerLimitTransitionRegionWidthUnits=m  UpperLimitSpecify=on  UpperLimitBound=pingyiup  UpperLimitBoundUnits=m  UpperLimitStiffness=sprsti  UpperLimitStiffnessUnits=N/m  UpperLimitDamping=damcoe  UpperLimitDampingUnits=N/(m/s)  UpperLimitTransitionRegionWidth=trare  UpperLimitTransitionRegionWidthUnits=m  PositionTargetSpecify=on  PositionTargetPriority=High  PositionTargetValue=spt  PositionTargetValueUnits=m  VelocityTargetSpecify=off  VelocityTargetPriority=Low  VelocityTargetValue=0.290646718208530  VelocityTargetValueUnits=m/s
  p1 : PMIOPort  Side=Right
  v1 : PMIOPort  Port=2  Side=Right
  a1 : PMIOPort  Port=3  Side=Right
  f1 : PMIOPort  Port=4  Side=Right
  Conn5 : PMIOPort  Port=5  Side=Left
  Conn6 : PMIOPort  Port=6  Side=Right
  L1 : PMIOPort  Port=7  Side=Left
  connections:
  Conn5/RConn1 -- B1/LConn1
  L1/RConn1 -- Prismatic Joint/LConn2
  B1/RConn1 -- Prismatic Joint/LConn1
  "\tT1"/LConn1 -- Prismatic Joint/RConn1
  Prismatic Joint/RConn5 -- f1/RConn1
  Conn6/RConn1 -- "\tT1"/RConn1
  Prismatic Joint/RConn2 -- p1/RConn1
  Prismatic Joint/RConn3 -- v1/RConn1
  Prismatic Joint/RConn4 -- a1/RConn1

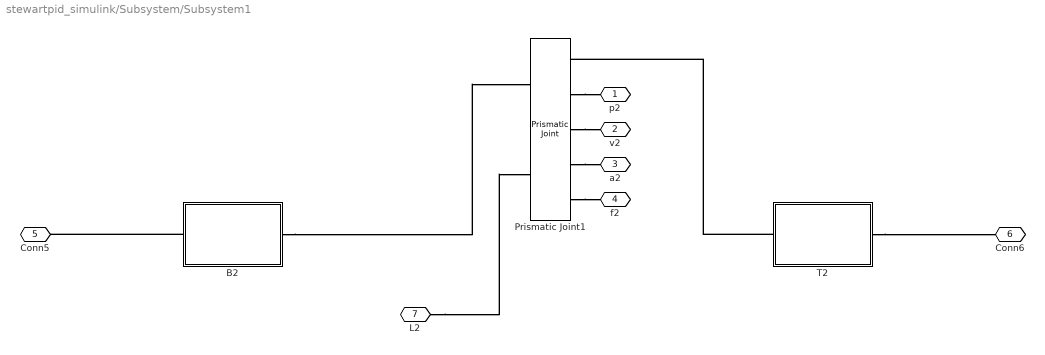
== system stewartpid_simulink/Subsystem/Subsystem1 ==
  "\tT2" : Subsystem
  B2 : Subsystem
  Prismatic Joint1 : sm_lib/Joints/Prismatic Joint  JointMode=Normal  SenseConstraintForce=off  SenseConstraintForceX=off  SenseConstraintForceY=off  SenseConstraintForceZ=off  SenseConstraintTorque=off  SenseConstraintTorqueX=off  SenseConstraintTorqueY=off  SenseConstraintTorqueZ=off  SenseTotalForce=off  SenseTotalForceX=off  SenseTotalForceY=off  SenseTotalForceZ=off  SenseTotalTorque=off  SenseTotalTorqueX=off  SenseTotalTorqueY=off  SenseTotalTorqueZ=off  CompositeWrenchDir=FollowerOnBase  CompositeWrenchFrame=BaseFrame  EquilibriumPosition=0  EquilibriumPositionUnits=m  SpringStiffness=0  SpringStiffnessUnits=N/m  DampingCoefficient=0  DampingCoefficientUnits=N/(m/s)  TorqueActuationMode=ComputedTorque  MotionActuationMode=InputMotion  SensePosition=on  SenseVelocity=on  SenseAcceleration=on  SenseTorqueForce=on  SenseLowerLimitTorqueForce=off  SenseUpperLimitTorqueForce=off  LowerLimitSpecify=on  LowerLimitBound=pingyilow  LowerLimitBoundUnits=m  LowerLimitStiffness=sprsti  LowerLimitStiffnessUnits=N/m  LowerLimitDamping=damcoe  LowerLimitDampingUnits=N/(m/s)  LowerLimitTransitionRegionWidth=trare  LowerLimitTransitionRegionWidthUnits=m  UpperLimitSpecify=on  UpperLimitBound=pingyiup  UpperLimitBoundUnits=m  UpperLimitStiffness=sprsti  UpperLimitStiffnessUnits=N/m  UpperLimitDamping=damcoe  UpperLimitDampingUnits=N/(m/s)  UpperLimitTransitionRegionWidth=trare  UpperLimitTransitionRegionWidthUnits=m  PositionTargetSpecify=on  PositionTargetPriority=High  PositionTargetValue=spt  PositionTargetValueUnits=m  VelocityTargetSpecify=off  VelocityTargetPriority=Low  VelocityTargetValue=0.092256794915314  VelocityTargetValueUnits=m/s
  p2 : PMIOPort  Side=Right
  v2 : PMIOPort  Port=2  Side=Right
  a2 : PMIOPort  Port=3  Side=Right
  f2 : PMIOPort  Port=4  Side=Right
  Conn5 : PMIOPort  Port=5  Side=Left
  Conn6 : PMIOPort  Port=6  Side=Right
  L2 : PMIOPort  Port=7  Side=Left
  connections:
  Prismatic Joint1/RConn5 -- f2/RConn1
  L2/RConn1 -- Prismatic Joint1/LConn2
  Prismatic Joint1/RConn4 -- a2/RConn1
  B2/RConn1 -- Prismatic Joint1/LConn1
  "\tT2"/LConn1 -- Prismatic Joint1/RConn1
  "\tT2"/RConn1 -- Conn6/RConn1
  B2/LConn1 -- Conn5/RConn1
  Prismatic Joint1/RConn3 -- v2/RConn1
  Prismatic Joint1/RConn2 -- p2/RConn1

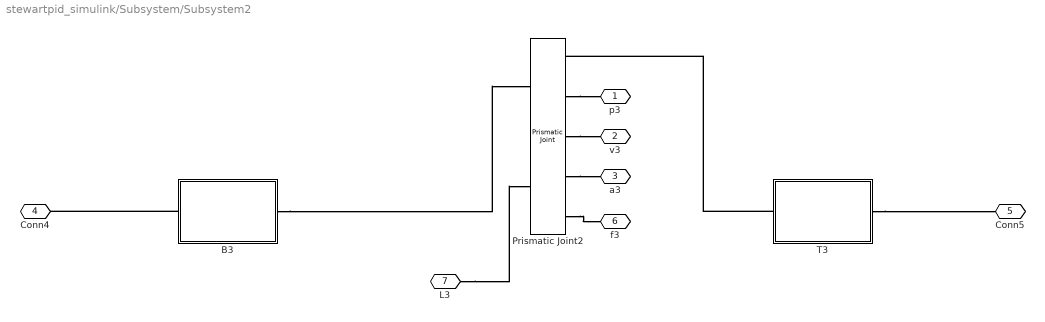
== system stewartpid_simulink/Subsystem/Subsystem2 ==
  "\tT3" : Subsystem
  B3 : Subsystem
  Prismatic Joint2 : sm_lib/Joints/Prismatic Joint  JointMode=Normal  SenseConstraintForce=off  SenseConstraintForceX=off  SenseConstraintForceY=off  SenseConstraintForceZ=off  SenseConstraintTorque=off  SenseConstraintTorqueX=off  SenseConstraintTorqueY=off  SenseConstraintTorqueZ=off  SenseTotalForce=off  SenseTotalForceX=off  SenseTotalForceY=off  SenseTotalForceZ=off  SenseTotalTorque=off  SenseTotalTorqueX=off  SenseTotalTorqueY=off  SenseTotalTorqueZ=off  CompositeWrenchDir=FollowerOnBase  CompositeWrenchFrame=BaseFrame  EquilibriumPosition=0  EquilibriumPositionUnits=m  SpringStiffness=0  SpringStiffnessUnits=N/m  DampingCoefficient=0  DampingCoefficientUnits=N/(m/s)  TorqueActuationMode=ComputedTorque  MotionActuationMode=InputMotion  SensePosition=on  SenseVelocity=on  SenseAcceleration=on  SenseTorqueForce=on  SenseLowerLimitTorqueForce=off  SenseUpperLimitTorqueForce=off  LowerLimitSpecify=on  LowerLimitBound=pingyilow  LowerLimitBoundUnits=m  LowerLimitStiffness=sprsti  LowerLimitStiffnessUnits=N/m  LowerLimitDamping=damcoe  LowerLimitDampingUnits=N/(m/s)  LowerLimitTransitionRegionWidth=trare  LowerLimitTransitionRegionWidthUnits=m  UpperLimitSpecify=on  UpperLimitBound=pingyiup  UpperLimitBoundUnits=m  UpperLimitStiffness=sprsti  UpperLimitStiffnessUnits=N/m  UpperLimitDamping=damcoe  UpperLimitDampingUnits=N/(m/s)  UpperLimitTransitionRegionWidth=trare  UpperLimitTransitionRegionWidthUnits=m  PositionTargetSpecify=on  PositionTargetPriority=High  PositionTargetValue=spt  PositionTargetValueUnits=m  VelocityTargetSpecify=off  VelocityTargetPriority=Low  VelocityTargetValue=0.929225656002702  VelocityTargetValueUnits=m/s
  p3 : PMIOPort  Side=Right
  v3 : PMIOPort  Port=2  Side=Right
  a3 : PMIOPort  Port=3  Side=Right
  Conn4 : PMIOPort  Port=4  Side=Left
  Conn5 : PMIOPort  Port=5  Side=Right
  f3 : PMIOPort  Port=6  Side=Right
  L3 : PMIOPort  Port=7  Side=Left
  connections:
  B3/LConn1 -- Conn4/RConn1
  B3/RConn1 -- Prismatic Joint2/LConn1
  "\tT3"/LConn1 -- Prismatic Joint2/RConn1
  Prismatic Joint2/RConn2 -- p3/RConn1
  Prismatic Joint2/RConn4 -- a3/RConn1
  L3/RConn1 -- Prismatic Joint2/LConn2
  "\tT3"/RConn1 -- Conn5/RConn1
  Prismatic Joint2/RConn3 -- v3/RConn1
  Prismatic Joint2/RConn5 -- f3/RConn1

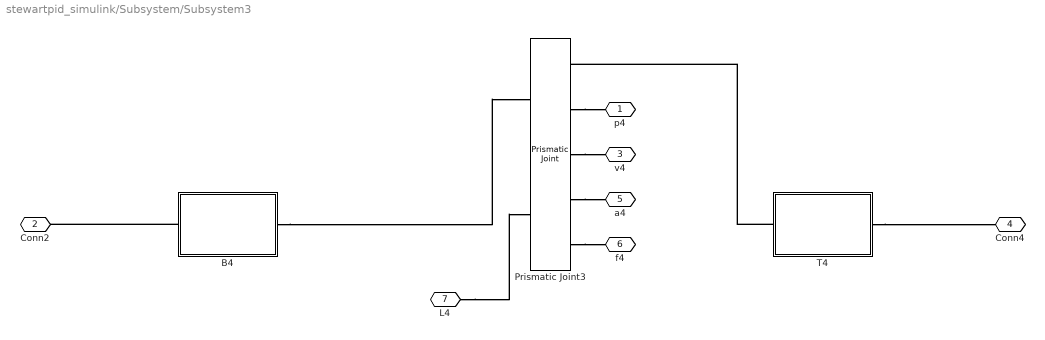
== system stewartpid_simulink/Subsystem/Subsystem3 ==
  "\tT4" : Subsystem
  B4 : Subsystem
  Prismatic Joint3 : sm_lib/Joints/Prismatic Joint  JointMode=Normal  SenseConstraintForce=off  SenseConstraintForceX=off  SenseConstraintForceY=off  SenseConstraintForceZ=off  SenseConstraintTorque=off  SenseConstraintTorqueX=off  SenseConstraintTorqueY=off  SenseConstraintTorqueZ=off  SenseTotalForce=off  SenseTotalForceX=off  SenseTotalForceY=off  SenseTotalForceZ=off  SenseTotalTorque=off  SenseTotalTorqueX=off  SenseTotalTorqueY=off  SenseTotalTorqueZ=off  CompositeWrenchDir=FollowerOnBase  CompositeWrenchFrame=BaseFrame  EquilibriumPosition=0  EquilibriumPositionUnits=m  SpringStiffness=0  SpringStiffnessUnits=N/m  DampingCoefficient=0  DampingCoefficientUnits=N/(m/s)  TorqueActuationMode=ComputedTorque  MotionActuationMode=InputMotion  SensePosition=on  SenseVelocity=on  SenseAcceleration=on  SenseTorqueForce=on  SenseLowerLimitTorqueForce=off  SenseUpperLimitTorqueForce=off  LowerLimitSpecify=on  LowerLimitBound=pingyilow  LowerLimitBoundUnits=m  LowerLimitStiffness=sprsti  LowerLimitStiffnessUnits=N/m  LowerLimitDamping=damcoe  LowerLimitDampingUnits=N/(m/s)  LowerLimitTransitionRegionWidth=trare  LowerLimitTransitionRegionWidthUnits=m  UpperLimitSpecify=on  UpperLimitBound=pingyiup  UpperLimitBoundUnits=m  UpperLimitStiffness=sprsti  UpperLimitStiffnessUnits=N/m  UpperLimitDamping=damcoe  UpperLimitDampingUnits=N/(m/s)  UpperLimitTransitionRegionWidth=trare  UpperLimitTransitionRegionWidthUnits=m  PositionTargetSpecify=on  PositionTargetPriority=High  PositionTargetValue=spt  PositionTargetValueUnits=m  VelocityTargetSpecify=off  VelocityTargetPriority=Low  VelocityTargetValue=1.031772065129790  VelocityTargetValueUnits=m/s
  p4 : PMIOPort  Side=Right
  Conn2 : PMIOPort  Port=2  Side=Left
  v4 : PMIOPort  Port=3  Side=Right
  Conn4 : PMIOPort  Port=4  Side=Right
  a4 : PMIOPort  Port=5  Side=Right
  f4 : PMIOPort  Port=6  Side=Right
  L4 : PMIOPort  Port=7  Side=Left
  connections:
  "\tT4"/LConn1 -- Prismatic Joint3/RConn1
  Prismatic Joint3/RConn5 -- f4/RConn1
  Prismatic Joint3/RConn3 -- v4/RConn1
  Prismatic Joint3/RConn4 -- a4/RConn1
  B4/RConn1 -- Prismatic Joint3/LConn1
  B4/LConn1 -- Conn2/RConn1
  L4/RConn1 -- Prismatic Joint3/LConn2
  "\tT4"/RConn1 -- Conn4/RConn1
  Prismatic Joint3/RConn2 -- p4/RConn1

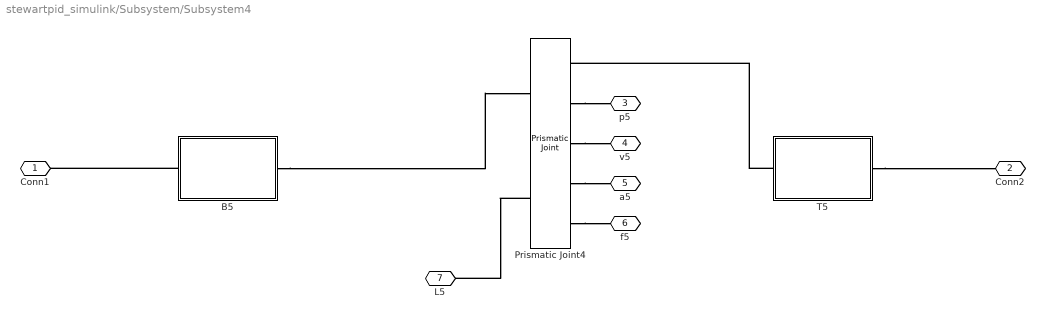
== system stewartpid_simulink/Subsystem/Subsystem4 ==
  "\tT5" : Subsystem
  B5 : Subsystem
  Prismatic Joint4 : sm_lib/Joints/Prismatic Joint  JointMode=Normal  SenseConstraintForce=off  SenseConstraintForceX=off  SenseConstraintForceY=off  SenseConstraintForceZ=off  SenseConstraintTorque=off  SenseConstraintTorqueX=off  SenseConstraintTorqueY=off  SenseConstraintTorqueZ=off  SenseTotalForce=off  SenseTotalForceX=off  SenseTotalForceY=off  SenseTotalForceZ=off  SenseTotalTorque=off  SenseTotalTorqueX=off  SenseTotalTorqueY=off  SenseTotalTorqueZ=off  CompositeWrenchDir=FollowerOnBase  CompositeWrenchFrame=BaseFrame  EquilibriumPosition=0  EquilibriumPositionUnits=m  SpringStiffness=0  SpringStiffnessUnits=N/m  DampingCoefficient=0  DampingCoefficientUnits=N/(m/s)  TorqueActuationMode=ComputedTorque  MotionActuationMode=InputMotion  SensePosition=on  SenseVelocity=on  SenseAcceleration=on  SenseTorqueForce=on  SenseLowerLimitTorqueForce=off  SenseUpperLimitTorqueForce=off  LowerLimitSpecify=on  LowerLimitBound=pingyilow  LowerLimitBoundUnits=m  LowerLimitStiffness=sprsti  LowerLimitStiffnessUnits=N/m  LowerLimitDamping=damcoe  LowerLimitDampingUnits=N/(m/s)  LowerLimitTransitionRegionWidth=trare  LowerLimitTransitionRegionWidthUnits=m  UpperLimitSpecify=on  UpperLimitBound=pingyiup  UpperLimitBoundUnits=m  UpperLimitStiffness=sprsti  UpperLimitStiffnessUnits=N/m  UpperLimitDamping=damcoe  UpperLimitDampingUnits=N/(m/s)  UpperLimitTransitionRegionWidth=trare  UpperLimitTransitionRegionWidthUnits=m  PositionTargetSpecify=on  PositionTargetPriority=High  PositionTargetValue=spt  PositionTargetValueUnits=m  VelocityTargetSpecify=off  VelocityTargetPriority=Low  VelocityTargetValue=0.363790525351351  VelocityTargetValueUnits=m/s
  Conn1 : PMIOPort  Side=Left
  Conn2 : PMIOPort  Port=2  Side=Right
  p5 : PMIOPort  Port=3  Side=Right
  v5 : PMIOPort  Port=4  Side=Right
  a5 : PMIOPort  Port=5  Side=Right
  f5 : PMIOPort  Port=6  Side=Right
  L5 : PMIOPort  Port=7  Side=Left
  connections:
  "\tT5"/LConn1 -- Prismatic Joint4/RConn1
  Prismatic Joint4/RConn5 -- f5/RConn1
  B5/RConn1 -- Prismatic Joint4/LConn1
  Prismatic Joint4/RConn4 -- a5/RConn1
  "\tT5"/RConn1 -- Conn2/RConn1
  Prismatic Joint4/RConn3 -- v5/RConn1
  Prismatic Joint4/RConn2 -- p5/RConn1
  B5/LConn1 -- Conn1/RConn1
  Prismatic Joint4/LConn2 -- L5/RConn1

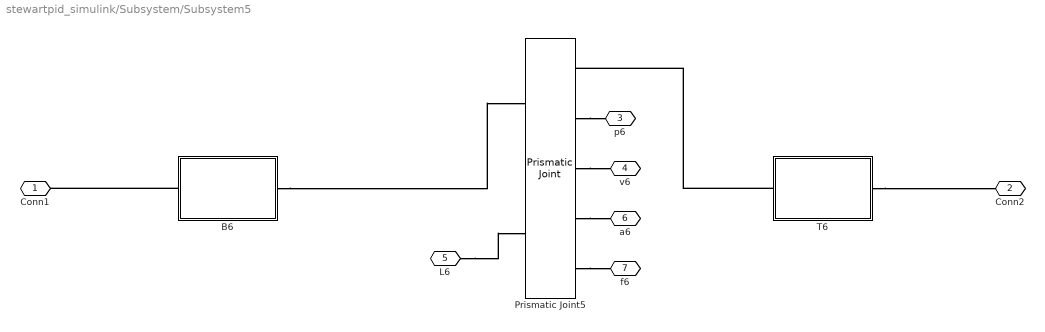
== system stewartpid_simulink/Subsystem/Subsystem5 ==
  "\tT6" : Subsystem
  B6 : Subsystem
  Prismatic Joint5 : sm_lib/Joints/Prismatic Joint  JointMode=Normal  SenseConstraintForce=off  SenseConstraintForceX=off  SenseConstraintForceY=off  SenseConstraintForceZ=off  SenseConstraintTorque=off  SenseConstraintTorqueX=off  SenseConstraintTorqueY=off  SenseConstraintTorqueZ=off  SenseTotalForce=off  SenseTotalForceX=off  SenseTotalForceY=off  SenseTotalForceZ=off  SenseTotalTorque=off  SenseTotalTorqueX=off  SenseTotalTorqueY=off  SenseTotalTorqueZ=off  CompositeWrenchDir=FollowerOnBase  CompositeWrenchFrame=BaseFrame  EquilibriumPosition=0  EquilibriumPositionUnits=m  SpringStiffness=0  SpringStiffnessUnits=N/m  DampingCoefficient=0  DampingCoefficientUnits=N/(m/s)  TorqueActuationMode=ComputedTorque  MotionActuationMode=InputMotion  SensePosition=on  SenseVelocity=on  SenseAcceleration=on  SenseTorqueForce=on  SenseLowerLimitTorqueForce=off  SenseUpperLimitTorqueForce=off  LowerLimitSpecify=on  LowerLimitBound=pingyilow  LowerLimitBoundUnits=m  LowerLimitStiffness=sprsti  LowerLimitStiffnessUnits=N/m  LowerLimitDamping=damcoe  LowerLimitDampingUnits=N/(m/s)  LowerLimitTransitionRegionWidth=trare  LowerLimitTransitionRegionWidthUnits=m  UpperLimitSpecify=on  UpperLimitBound=pingyiup  UpperLimitBoundUnits=m  UpperLimitStiffness=sprsti  UpperLimitStiffnessUnits=N/m  UpperLimitDamping=damcoe  UpperLimitDampingUnits=N/(m/s)  UpperLimitTransitionRegionWidth=trare  UpperLimitTransitionRegionWidthUnits=m  PositionTargetSpecify=on  PositionTargetPriority=High  PositionTargetValue=spt  PositionTargetValueUnits=m  VelocityTargetSpecify=off  VelocityTargetPriority=Low  VelocityTargetValue=0.083220054818936  VelocityTargetValueUnits=m/s
  Conn1 : PMIOPort  Side=Left
  Conn2 : PMIOPort  Port=2  Side=Right
  p6 : PMIOPort  Port=3  Side=Right
  v6 : PMIOPort  Port=4  Side=Right
  L6 : PMIOPort  Port=5  Side=Left
  a6 : PMIOPort  Port=6  Side=Right
  f6 : PMIOPort  Port=7  Side=Right
  connections:
  B6/RConn1 -- Prismatic Joint5/LConn1
  "\tT6"/RConn1 -- Conn2/RConn1
  "\tT6"/LConn1 -- Prismatic Joint5/RConn1
  B6/LConn1 -- Conn1/RConn1
  Prismatic Joint5/RConn2 -- p6/RConn1
  Prismatic Joint5/RConn5 -- f6/RConn1
  L6/RConn1 -- Prismatic Joint5/LConn2
  Prismatic Joint5/RConn3 -- v6/RConn1
  Prismatic Joint5/RConn4 -- a6/RConn1
